simulink model "MCU_vectorControl_Simulation"  (R2024a)
settings: Solver=ode3  StartTime=0.0  StopTime=3  FixedStep=Ts  MaxStep=1e-4  RelTol=1e-3  EnableMultiTasking=on
values from neighbouring files (symbols this model uses):
  Ts = 1e-4    (= 0.0001)    [MCU_initVectorControlParameters.m]
undefined symbols (not defined in the file or in its folder): control, DiscIntNeverNeededParam, dspic33CK, insa_motormodel, inverter, LVMC, motor, NumBits1, NumBits2, PMSM, PosRange1, PosRange2, Slope1, Slope2
libraries: simulink x22, embmathops x1
(part 1 of 2)
Description:
  | Motor Control Simulation Demo
  | contacts : romain.delpoux@insa-lyon.fr, lubin.kerhuel@microchip.com
settings Model: DSRTSU_INTERNAL_RTI_VER=470  DSRTSU_INTERNAL_RTI_TYPE=rti1104  DSRTSU_INTERNAL_RTIFPGA=60  Creator=rdelpoux  LastModifiedBy=rdelpoux
settings SolverCC: ZeroCrossControl=DisableAll  AlgebraicLoopSolver=TrustRegion
settings DataIOCC: LimitDataPoints=on  SaveFormat=Array  ReturnWorkspaceOutputs=off
settings OptimizationCC: BlockReduction=off  OptimizeBlockIOStorage=off  BufferReuse=off  ReuseModelBlockBuffer=off  GlobalBufferReuse=off  ExpressionFolding=off  LocalBlockOutputs=off  LifeSpan=inf  OptimizeDataStoreBuffers=off  BusAssignmentInplaceUpdate=off
settings DebuggingCC: SolverPrmCheckMsg=warning  MultiTaskDSMMsg=none  UnconnectedInputMsg=warning  UnconnectedOutputMsg=warning  UnconnectedLineMsg=warning  SFUnexpectedBacktrackingDiag=warning  SFNoUnconditionalDefaultTransitionDiag=warning  SFExecutionAtInitializationDiag=none  ArithmeticOperatorsInVariantConditions=warning
settings HardwareCC: ProdBitPerPointer=32  ProdBitPerSizeT=32  ProdBitPerPtrDiffT=32  ProdLargestAtomicInteger=Integer  ProdEndianess=BigEndian  ProdWordSize=32  ProdHWDeviceType=Generic->Custom  TargetIntDivRoundTo=Zero  TargetEndianess=BigEndian  TargetHWDeviceType=Generic->Custom
settings ModelReferenceCC: EnableRefExpFcnMdlSchedulingChecks=on  PropagateSignalLabelsOutOfModel=off
settings SFSimCC: SimUseLocalCustomCode=off  CustomCodeUndefinedFunction=UseInterfaceOnly
settings RTWCC: Description=dSPACE DS1104 Hardware Platform  SystemTargetFile=rti1104.tlc  MakeCommand=make_rti  TemplateMakefile=rti1104.tmf  RTWUseLocalCustomCode=off  GPUComputeCapability=3.5  DLArmComputeVersion=19.05
settings CodeAppCC: StateflowObjectComments=on
settings STFCustomTargetCC: TargetLangStandard=C89/C90 (ANSI)  ParMdlRefBuildCompliant=on  MatFileLogging=on  UseToolchainInfoCompliant=off  SystemTargetFile=rti1104.tlc
settings GRTTargetCC: TargetLangStandard=C89/C90 (ANSI)  CompOptLevelCompliant=off  ConcurrentExecutionCompliant=off  CombineOutputUpdateFcns=off  CPPClassGenCompliant=off  GRTInterface=on  UseToolchainInfoCompliant=off  ExtModeMexFile=noextcomm
settings ConfigComp: CovMetricSettings=dw  CovSaveCumulativeToWorkspaceVar=on  CovSaveSingleToWorkspaceVar=on  CovExternalEMLEnable=off  CovSFcnEnable=off

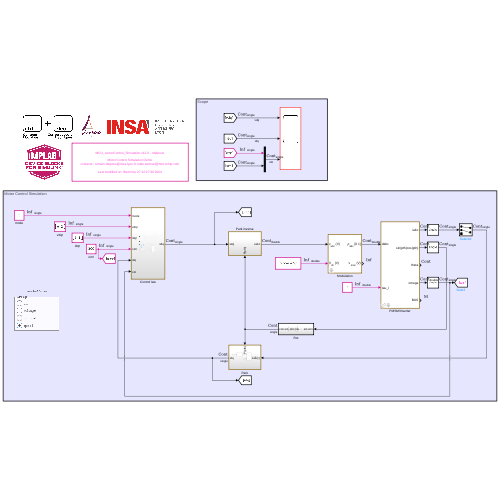
[thumbnail: Simulink's stored preview of the top-level diagram]
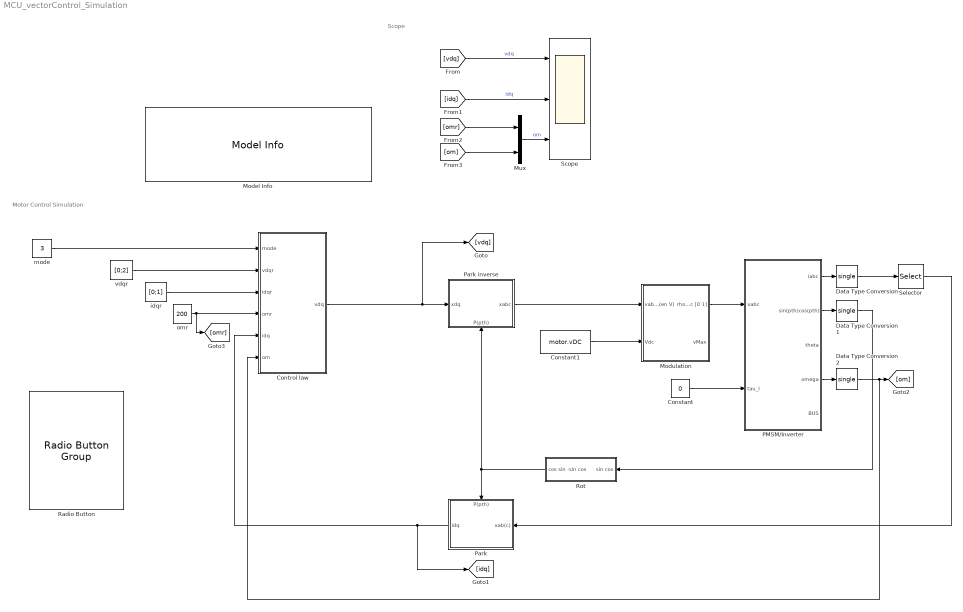
== system MCU_vectorControl_Simulation ==
  note: Scope
  note: Motor Control Simulation
  Constant : Constant  Value=0
  Constant1 : Constant  Value=motor.vDC
  Control law : Subsystem
      settings: LibrarySourceBlock=insa_control_base/Control law
  Data Type Conversion : DataTypeConversion  OutDataTypeStr=single  SaturateOnIntegerOverflow=off  RndMeth=Floor
  Data Type Conversion1 : DataTypeConversion  OutDataTypeStr=single  SaturateOnIntegerOverflow=off  RndMeth=Floor
  Data Type Conversion2 : DataTypeConversion  OutDataTypeStr=single  SaturateOnIntegerOverflow=off  RndMeth=Floor
  Model Info : simulink/Model-Wide Utilities/Model Info  Frame=on  DisplayStringWithTags=|  HorizontalTextAlignment=Center  LeftAlignmentValue=0.5
      | %<ModelName> v%<ModelVersion> - %<Creator>
      | 
      | %<Description>
      | 
      | Last modified on: %<LastModificationDate>
  Modulation : Subsystem  mask{modulation=Space Vector, mod=0}
      mask init:
      | switch modulation
      |     case 'Sinusoidale'
      |         mod = 0;
      |     otherwise
      |         mod = 1;
      | end
      mask TypeOptions modulation: Sinusoidale | Space Vector
      mask DialogControl DescGroupVar Prompt: Modulation interssecticve
      mask DialogControl DescTextVar Prompt: Choose between sinus or space vector modulation
      mask Display:
      | port_label('output', 1, '\rho_{abc} [0 1]', 'texmode','on')
      | port_label('output', 2, 'v_{\rm max} (V)', 'texmode','on')
      | port_label('input', 1, 'v_{abc} (V)', 'texmode','on')
      | port_label('input', 2, 'V_{dc} (V)', 'texmode','on')
  Mux : Mux  Inputs=2
  PMSM/Inverter : Subsystem  AncestorBlock=insa_motormodel/PMSM  mask(Test){presetMotor=Teknic-2310P, modelPMSM=Teknic-2310P, p=4, R=0.656, L=0.00035, Phif=0.0066, J=1e-05, F=1e-05, C0=0.01, omegaMax=350, encoderLines=1000, enableInverter=on, presetInverter=LVMC (DM330031), modelInverter=dspic33CK-LVMC, Vdc=24, iMax=10, FPWM=20000, PWMmax=5000, enableDTcomp=off, dT=1, ADCbits=12, ADCgainCurr=21.83, ADCgainVolt=69.3, Ts=1e-4}
      mask prompts: presetMotor "Pre Defined Motor"; modelPMSM "PMSM model"; p "Pole pairs p"; R "Phase resistor R (Ohm)"; L "Phase inductance L (H)"; Phif "Flux constant Phif (Wb)"; J "Inertia J (kg.m^2)"; F "Damping coefficient F (N.m.s/rad)"; C0 "Coulomb friction C0 (N.m)"; omegaMax "Max Speed (rad/s)"; encoderLines "lines"; enableInverter "Enable"; presetInverter "Pre Defined Inverter"; modelInverter "Inverter Model"; Vdc "DC Voltage Vdc (V)"; iMax "Max Current iMax (A)"; FPWM "PWM frequency"; enableDTcomp "Dead time Compensation"; dT "Dead time (us)"; ADCbits "Precision (bits)"; ADCgainCurr "Currents gain"; ADCgainVolt "Voltage gain"; Ts "Ts (s)"
      mask init:
      | % Mototor definition
      | pmsm = struct;
      | switch presetMotor
      |     case 'Teknic-2310P'
      |         pmsm.modelPMSM    = 'Teknic-2310P';                                     %           // Manufacturer Model Number
      |         pmsm.p        = 4;                                                  %           // Pole Pairs for the motor
      |         pmsm.R        = 0.656;                                              %Ohm        // Stator Resistor
      |         pmsm.L        = 0.35e-3;                                            %H          // Inductance value
      |         pmsm.Phif     = 6.6e-3;                                             %Wb         // PM flux
      |         pmsm.J        = 1e-05;                                              %Kg-m2      // Inertia in SI units
      |         pmsm.F        = 1.e-05;                                             %Kg-m2/s    // Friction Co-efficient
      |         pmsm.C0       = 0.01;                                               %Kg-m2      // Dry friction
      |         pmsm.omegaMax    = 350;                                            %rad/spm    // Max speed
      |         pmsm.encoderLines = 1000;
      |     case 'Custom'
      |         pmsm.modelPMSM    = 'Custom';                                           %           // Manufacturer Model Number
      |         pmsm.p        = p;                                                  %           // Pole Pairs for the motor
      |         pmsm.R        = R;                                                  %Ohm        // Stator Resistor
      |         pmsm.L        = L;                                                  %H          // Inductance value
      |         pmsm.Phif     = Phif;                                               %Wb         // PM flux
      |         pmsm.J        = J;                                                  %Kg-m2      // Inertia in SI units
      |         pmsm.F        = F;                                                  %Kg-m2/s    // Friction Co-efficient
      |         pmsm.C0       = C0;                                                 %Kg-m2      // Dry friction
      |         pmsm.omegaMax    = omegaMax;                                             %rad/spm    // Max speed
      |         pmsm.encoderLines = encoderLines;
      | end
      | 
      | ff = fields(pmsm);
      | for i=1:numel(ff)
      |     set_param(gcb,ff{i},num2str(pmsm.(ff{i})) );
      | end
      | 
      | % switch presetMotor
      | %      case 'Custom'
      | %          set_param(gcb,model,(pmsm.model) );
      | %      otherwise 'Teknic-2310P'
      | %
      | %
      | % end
      | 
      | assignin('base','pmsm',pmsm);
      | 
      | % Inverter Definition
      | inverter = struct;
      | switch presetInverter
      |     case 'LVMC (DM330031)'
      |         inverter.modelInverter = 'dspic33CK-LVMC';
      |         inverter.vDC = 24;                          %V          // DC voltage
      |         inverter.iMax = 10;                         %A      	// Rated current (phase-peak)
      |         inverter.ADCbits = 12;                      %bits       // ADC precision
      |         inverter.ADCgainCurr = 21.83;                   %
      |         inverter.ADCgainVolt = 69.3;                   %
      |         inverter.PWMmax = 5000;
      |         inverter.dT = 1;                            %us         // Deat Time
      |         inverter.FPWM = 20e3;                       %Hz         // PWM frequency
      |     case 'MCLV2 (DM330021-2)'
      | end
      | 
      | ff = fields(inverter);
      | for i=1:numel(ff)
      |     set_param(gcb,ff{i},num2str(inverter.(ff{i})) );
      | end
      | assignin('base','inverter',inverter);
      | 
      | assignin('base','Ts',Ts);
      settings: LibrarySourceBlock=insa_motormodel/PMSM
      mask Help: disp('{\itEquation:}  \alpha^2 + \beta^2 \rightarrow \gamma^2, \chi, \phi_3 = {\bfcool}', 'texmode','on')
      mask TypeOptions presetMotor: Custom | Teknic-2310P | Short HURST (AC300020) | Long HURST (AC300022)
      mask TypeOptions presetInverter: Custom | LVMC (DM330031) | MCLV2 (DM330021-2)
      mask DialogControl DescGroupVar Prompt: Moteur Synchrone à aimants permanents
      mask DialogControl DescTextVar Prompt: PMSM Model
      mask DialogControl Container6 Prompt: Motor Parameters
      mask DialogControl Container3 Prompt: Electrical parameters
      mask DialogControl Container4 Prompt: Mecanical parameter
      mask DialogControl Container9 Prompt: Encoder
      mask DialogControl Container11 Prompt: Inverter
      mask DialogControl Container12 Prompt: Inverter Constraints
      mask DialogControl Container10 Prompt: PWM
      mask DialogControl Container8 Prompt: ADC
      mask DialogControl Container13 Prompt: Sample Time
      mask Display:
      | switch get_param(gcb,'enableInverter')
      |     case 'off'
      |     port_label('input', 1, 'vabc');
      |     case 'on'
      |     port_label('input', 1, 'dabc');
      | end
      | port_label('input', 2, 'tau_l');
      | 
      | port_label('output', 1, 'iabc');
      | port_label('output', 2, 'sin(pth)cos(pth)');
      | port_label('output', 3, 'theta');
      | port_label('output', 4, 'omega');
      | port_label('output', 5, 'BUS');
  Park : Subsystem
      settings: PortSchema="{\"entries\":[{\"content\":{\"sides\":[{\"content\":{\"connectorIds\":[\"In1\"]},\"type\":\"ConnectorPlacement.EquallySpacedRectSide\",\"uuid\":\"ebf2fcb8-f94c-4630-a735-fb74e68b604e\"},{\"content\":{\"connectorIds\":[\"Out1\"],\"side\":\"RIGHT\"},\"type\":\"ConnectorPlacement.EquallySpacedRectSide\",\"uuid\":\"fb89ad3f-9420-4065-992c-c6d77ce245e0\"},{\"content\":{\"connectorIds\":[\"In2\"],\"side\":\"TOP\"},\"type\":\"ConnectorPlacement.EquallySpacedRectSide\",\"uuid\":\"0249ceba-2241-48c9-87d4-d9d6f381f2d7\"}]},\"type\":\"ConnectorPlacement.EquallySpacedConnector\",\"uuid\":\"eecfd82d-5918-403e-a677-09fe1d8cc737\"}],\"packageUris\":[\"http://schema.mathworks.com/mf0/Connector/R2020b\"],\"version\":\"1.0\"}"
  Park inverse : Subsystem
      settings: PortSchema="{\"entries\":[{\"content\":{\"sides\":[{\"content\":{\"connectorIds\":[\"In1\"]},\"type\":\"ConnectorPlacement.EquallySpacedRectSide\",\"uuid\":\"4c11ef0a-1978-4a73-9b5c-4d5650fcee33\"},{\"content\":{\"connectorIds\":[\"Out1\"],\"side\":\"RIGHT\"},\"type\":\"ConnectorPlacement.EquallySpacedRectSide\",\"uuid\":\"28284572-70c7-45ef-9db5-4b5788e96454\"},{\"content\":{\"side\":\"TOP\"},\"type\":\"ConnectorPlacement.EquallySpacedRectSide\",\"uuid\":\"3a1fbce2-0868-491b-8e3a-2b3a7a0d615d\"},{\"content\":{\"connectorIds\":[\"In2\"],\"side\":\"BOTTOM\"},\"type\":\"ConnectorPlacement.EquallySpacedRectSide\",\"uuid\":\"e63426ef-821a-4774-a922-a3f70d9b2116\"}]},\"type\":\"ConnectorPlacement.EquallySpacedConnector\",\"uuid\":\"285593a5-8af6-47f2-83d9-d6ebce98de71\"}],\"packageUris\":[\"http://schema.mathworks.com/mf0/Connector/R2020b\"],\"version\":\"1.0\"}"
  Radio Button : RadioButtonGroup  SelectedLabel=speed  ButtonGroupName=Group
      settings: Values={{'off', 'voltage', 'current', 'speed'}, [0 1 2 3]}
  Rot : Subsystem
  Scope : Scope  NumInputPorts=3
  Selector : Selector  InputPortWidth=3  IndexOptions=Index vector (dialog)  Indices=[1 2]  OutputSizes=1
  idqr : Constant  Value=[0;1]  OutDataTypeStr=single
  mode : Constant  Value=3  OutDataTypeStr=single
  omr : Constant  Value=200  OutDataTypeStr=single
  vdqr : Constant  Value=[0;2]  OutDataTypeStr=single
  wires:
  [vdq] -> Scope/1  "vdq"
  [idq] -> Scope/2  "idq"
  [omr] -> Mux/1
  [om] -> Mux/2
  Mux/1 -> Scope/3  "om"
  Control law/1(vdq) -> [vdq], Park inverse/1(xdq)
  vdqr/1 -> Control law/2(vdqr)
  mode/1 -> Control law/1(mode)
  omr/1 -> Control law/4(omr), [omr]
  idqr/1 -> Control law/3(idqr)
  Constant/1 -> PMSM/Inverter/2(tau_l)
  PMSM/Inverter/1(iabc) -> Data Type Conversion/1
  Selector/1 -> Park/1(xab(c))
  PMSM/Inverter/2(sin(pth)cos(pth)) -> Data Type Conversion1/1
  Modulation/1(rho_abc [0 1]) -> PMSM/Inverter/1(xabc)
  PMSM/Inverter/4(omega) -> Data Type Conversion2/1
  Park/1(idq) -> Control law/5(idq), [idq]
  Data Type Conversion/1 -> Selector/1
  Data Type Conversion1/1 -> Rot/1(sin cos)
  Data Type Conversion2/1 -> Control law/6(om), [om]
  Constant1/1 -> Modulation/2(Vdc)
  Rot/1("cos sin -sin cos ") -> Park inverse/2(P(pth)), Park/2(P(pth))
  Park inverse/1(xabc) -> Modulation/1("vabc (en V) ")

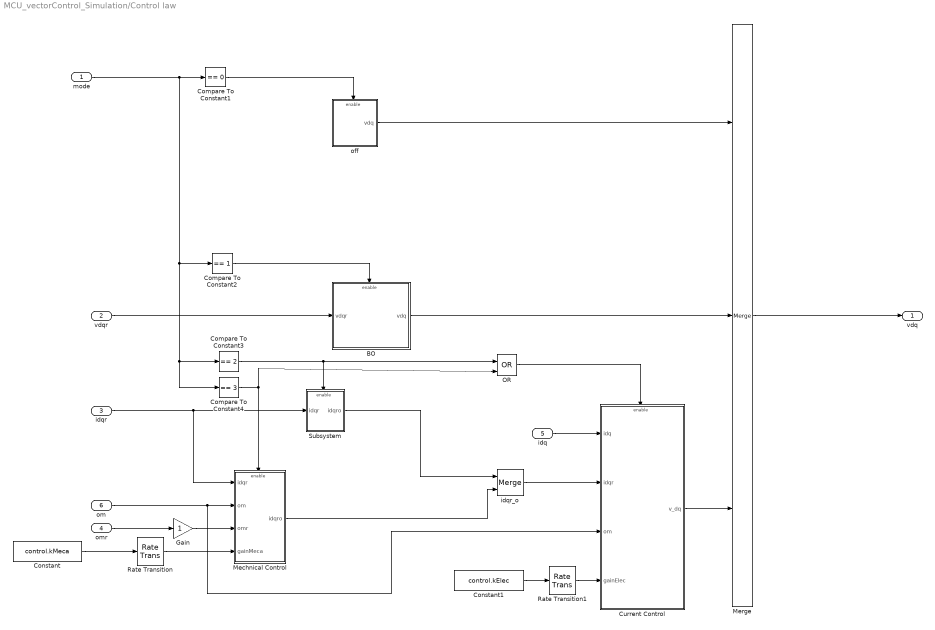
== system MCU_vectorControl_Simulation/Control law ==
  mode : Inport
  vdqr : Inport  Port=2
  idqr : Inport  Port=3
  omr : Inport  Port=4
  idq : Inport  Port=5
  om : Inport  Port=6
  BO : Subsystem
  Compare To Constant1 : simulink/Logic and Bit Operations/Compare To Constant  relop===  const=0  OutDataTypeStr=boolean
  Compare To Constant2 : simulink/Logic and Bit Operations/Compare To Constant  relop===  const=1  OutDataTypeStr=boolean
  Compare To Constant3 : simulink/Logic and Bit Operations/Compare To Constant  relop===  const=2  OutDataTypeStr=boolean
  Compare To Constant4 : simulink/Logic and Bit Operations/Compare To Constant  relop===  const=3  OutDataTypeStr=boolean
  Constant : Constant  Value=control.kMeca  OutDataTypeStr=single
  Constant1 : Constant  Value=control.kElec  OutDataTypeStr=double
  Current Control : Subsystem  AncestorBlock=insa_control_base/Current Control
      settings: LibrarySourceBlock=insa_control_base/Current Control
  Gain : Gain
  Mechnical Control : Subsystem
  Merge : Merge  Inputs=3
  OR : Logic  Operator=OR  IconShape=distinctive  AllPortsSameDT=off  OutDataTypeStr=boolean
  Rate Transition : RateTransition
  Rate Transition1 : RateTransition
  Subsystem : Subsystem
  idqr_o : Merge
  off : Subsystem
  vdq : Outport  VectorParamsAs1DForOutWhenUnconnected=off
  wires:
  omr/1 -> Gain/1
  idqr/1 -> Mechnical Control/1(idqr), Subsystem/1(idqr)
  vdqr/1 -> BO/1(vdqr)
  Current Control/1(v_dq) -> Merge/3
  idqr_o/1 -> Current Control/2(idqr)
  idq/1 -> Current Control/1(idq)
  OR/1 -> Current Control/Enable
  om/1 -> Current Control/3(om), Mechnical Control/2(om)
  Compare To Constant4/1 -> Mechnical Control/Enable, OR/2
  Mechnical Control/1(idqro) -> idqr_o/2
  Subsystem/1(idqro) -> idqr_o/1
  mode/1 -> Compare To Constant1/1, Compare To Constant4/1, Compare To Constant3/1, Compare To Constant2/1
  Compare To Constant3/1 -> Subsystem/Enable, OR/1
  Compare To Constant1/1 -> off/Enable
  off/1(vdq) -> Merge/1
  Compare To Constant2/1 -> BO/Enable
  BO/1(vdq) -> Merge/2
  Merge/1 -> vdq/1
  Constant/1 -> Rate Transition/1
  Constant1/1 -> Rate Transition1/1
  Rate Transition/1 -> Mechnical Control/4(gainMeca)
  Rate Transition1/1 -> Current Control/4(gainElec)
  Gain/1 -> Mechnical Control/3(omr)

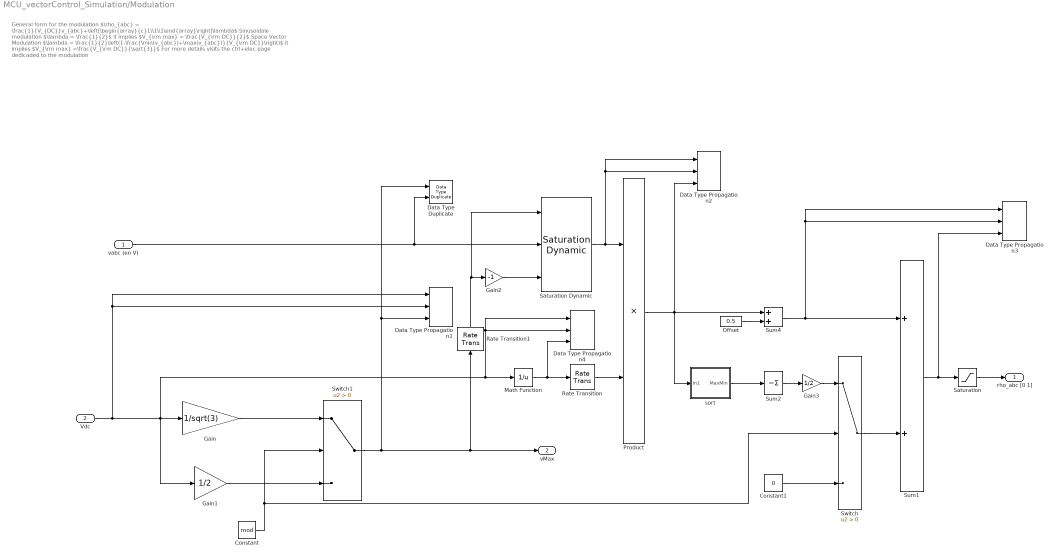
== system MCU_vectorControl_Simulation/Modulation ==
  note: General form for the modulation
      | $\rho_{abc} = \frac{1}{V_{DC}}v_{abc}+\left[\begin{array}{c}1\\1\\1\end{array}\right]\lambda$
      | Sinusoidale modulation
      | $\lambda = \frac{1}{2}$ it implies $V_{\rm max} = \frac{V_{\rm DC}}{2}$
      | Space Vector Modulation
      | $\lambda = \frac{1}{2}\left(1-\frac{\min(v_{abc})+\max(v_{abc})}{V_{\rm DC}}\right)$ it implies $V_{\rm max} =\frac{V_{\rm DC}}{\sqrt{3}}$
      | For more details visits the ctrl+elec page dedicaded to the modulation
  "vabc (en V) " : Inport
  Vdc : Inport  Port=2
  Constant : Constant  Value=mod  OutDataTypeStr=boolean
  Constant1 : Constant  Value=0  OutDataTypeStr=Inherit: Inherit via back propagation
  Data Type Duplicate : DataTypeDuplicate
  Data Type Propagation1 : simulink/Signal Attributes/Data Type Propagation  PropDataType=fixdt(1, 16)  IfRefDouble=double  IfRefSingle=single  IsSigned=TRUE  NumBitsBase=max([NumBits1 NumBits2])  NumBitsMult=1  NumBitsAdd=0  NumBitsAllowFinal=[1:128]  PropScaling=2^-(15-ceil(log2(inverter.vDC/sqrt(3))))  ValuesUsedBestPrec=[100 -100]  SlopeBase=max([PosRange1 PosRange2])  SlopeMult=1/sqrt(3)  SlopeAdd=0  BiasBase=Bias1  BiasMult=1  BiasAdd=0
  Data Type Propagation2 : simulink/Signal Attributes/Data Type Propagation  PropDataType=fixdt(1, 16)  IfRefDouble=double  IfRefSingle=single  IsSigned=TRUE  NumBitsBase=max([NumBits1 NumBits2])  NumBitsMult=1  NumBitsAdd=0  NumBitsAllowFinal=[1:128]  PropScalingMode=Specify via dialog  PropScaling=2^-14  ValuesUsedBestPrec=[100 -100]  SlopeBase=Slope1/Slope2  SlopeMult=1  SlopeAdd=0  BiasBase=Bias1  BiasMult=1  BiasAdd=0
  Data Type Propagation3 : simulink/Signal Attributes/Data Type Propagation  PropDataType=fixdt(1, 16)  IfRefDouble=double  IfRefSingle=single  IsSigned=FALSE  NumBitsBase=max([NumBits1 NumBits2])  NumBitsMult=1  NumBitsAdd=0  NumBitsAllowFinal=[1:128]  PropScalingMode=Specify via dialog  PropScaling=2^-14  ValuesUsedBestPrec=[100 -100]  SlopeBase=Slope1/Slope2  SlopeMult=1  SlopeAdd=0  BiasBase=Bias1  BiasMult=1  BiasAdd=0
  Data Type Propagation4 : simulink/Signal Attributes/Data Type Propagation  PropDataType=fixdt(1, 16)  IfRefDouble=double  IfRefSingle=single  IsSigned=FALSE  NumBitsBase=max([NumBits1 NumBits2])  NumBitsMult=1  NumBitsAdd=0  NumBitsAllowFinal=[1:128]  PropScalingMode=Specify via dialog  PropScaling=2^-16  ValuesUsedBestPrec=[100 -100]  SlopeBase=max([PosRange1 PosRange2])  SlopeMult=1/sqrt(3)  SlopeAdd=0  BiasBase=Bias1  BiasMult=1  BiasAdd=0
  Gain : Gain  Gain=1/sqrt(3)  OutDataTypeStr=Inherit: Same as input
  Gain1 : Gain  Gain=1/2  OutDataTypeStr=Inherit: Same as input
  Gain2 : Gain  Gain=-1  ParamDataTypeStr=int16  OutDataTypeStr=Inherit: Inherit via back propagation
  Gain3 : Gain  Gain=1/2  OutDataTypeStr=Inherit: Same as input
  Math Function : Math  Operator=reciprocal  OutputSignalType=real  OutDataTypeStr=Inherit: Inherit via back propagation  SaturateOnIntegerOverflow=off
  "Offset " : Constant  Value=0.5  OutMin=[0]  OutMax=[1]  OutDataTypeStr=Inherit: Inherit via back propagation
  Product : Product  Inputs=**  OutDataTypeStr=Inherit: Inherit via back propagation  SaturateOnIntegerOverflow=on
  Rate Transition : RateTransition
  Rate Transition1 : RateTransition
  Saturation : Saturate  UpperLimit=1  LowerLimit=0
  Saturation Dynamic : simulink/Discontinuities/Saturation Dynamic  OutMin=[]  OutMax=[]  OutDataTypeStr=Inherit: Same as second input  OutDataType=fixdt(1, 16)  OutScaling=2^-10  DoSatur=off
  Sum1 : Sum  OutMin=[0]  OutMax=[1]  OutDataTypeStr=Inherit: Inherit via back propagation  InputSameDT=on  SaturateOnIntegerOverflow=on
  Sum2 : Sum  Inputs=-  OutMin=[-1]  OutMax=[1]  InputSameDT=on  SaturateOnIntegerOverflow=on  OutDataTypeStr=Inherit: Same as first input
  Sum4 : Sum  OutMin=[-1]  OutMax=[1]  InputSameDT=on  SaturateOnIntegerOverflow=on  OutDataTypeStr=Inherit: Same as first input
  Switch : Switch  Criteria=u2 > Threshold  SaturateOnIntegerOverflow=off  InputSameDT=off
  Switch1 : Switch  Criteria=u2 > Threshold  OutDataTypeStr=Inherit: Inherit via back propagation  SaturateOnIntegerOverflow=off  InputSameDT=off
  sort : Subsystem
  rho_abc [0 1] : Outport  VectorParamsAs1DForOutWhenUnconnected=off
  vMax : Outport  Port=2  VectorParamsAs1DForOutWhenUnconnected=off
  wires:
  Sum1/1 -> Saturation/1, Data Type Propagation3/3
  Vdc/1 -> Data Type Propagation1/2, Data Type Propagation1/1, Gain/1, Math Function/1, Data Type Propagation4/2, Data Type Propagation4/1, Gain1/1
  Gain3/1 -> Switch/1
  Saturation/1 -> rho_abc [0 1]/1
  Saturation Dynamic/1 -> Product/1, Data Type Propagation2/1, Data Type Propagation2/2
  Gain1/1 -> Switch1/3
  Gain/1 -> Switch1/1
  sort/1(MaxMin) -> Sum2/1
  Sum2/1 -> Gain3/1
  Sum4/1 -> Data Type Propagation3/2, Data Type Propagation3/1, Sum1/1
  Constant1/1 -> Switch/3
  Switch/1 -> Sum1/2
  "Offset "/1 -> Sum4/2
  Product/1 -> Data Type Propagation2/3, Sum4/1, sort/1(In1)
  Gain2/1 -> Saturation Dynamic/3
  Math Function/1 -> Data Type Propagation4/3, Rate Transition/1
  Switch1/1 -> Rate Transition1/1, vMax/1, Data Type Propagation1/3, Data Type Duplicate/1
  Constant/1 -> Switch1/2, Switch/2
  "vabc (en V) "/1 -> Data Type Duplicate/2, Saturation Dynamic/2
  Rate Transition/1 -> Product/2
  Rate Transition1/1 -> Saturation Dynamic/1, Gain2/1

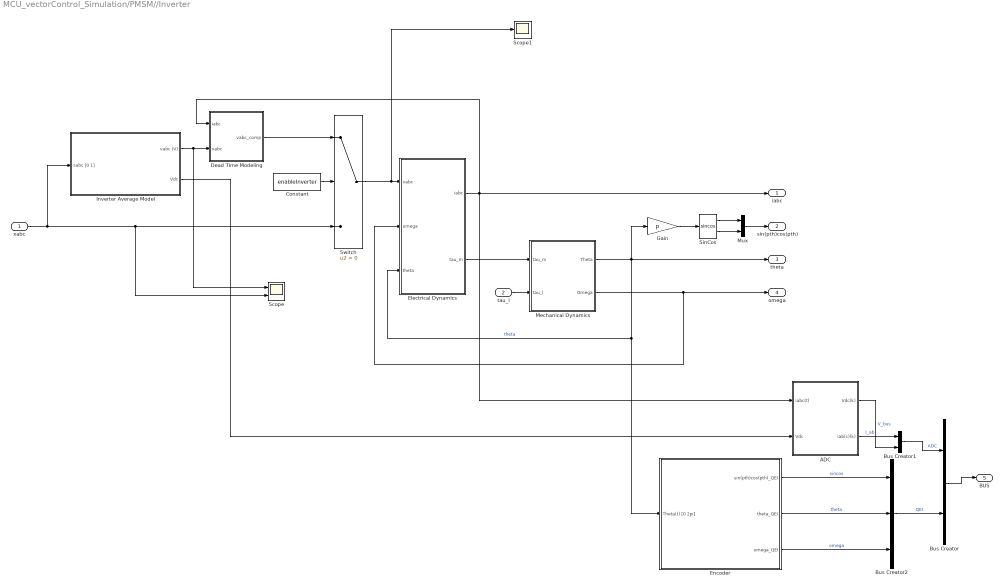
== system MCU_vectorControl_Simulation/PMSM//Inverter ==
  xabc : Inport
  tau_l : Inport  Port=2
  ADC : Subsystem
  Bus Creator : BusCreator  Inputs=2
  Bus Creator1 : BusCreator  Inputs=2
  Bus Creator2 : BusCreator  Inputs=3
  Constant : Constant  Value=enableInverter  OutDataTypeStr=boolean
  Dead Time Modeling : Subsystem
  Electrical Dynamics : Subsystem
  Encoder : Subsystem
  Gain : Gain  Gain=p
  Inverter Average Model : Subsystem
      settings: LibrarySourceBlock=insa_motormodel/Inverter Average Model
  Mechanical Dynamics : Subsystem
  Mux : Mux  Inputs=2
  Scope : Scope  NumInputPorts=2
  Scope1 : Scope
  SinCos : Trigonometry  Operator=sincos
  Switch : Switch  Criteria=u2 > Threshold  SaturateOnIntegerOverflow=off  InputSameDT=off
  iabc : Outport  VectorParamsAs1DForOutWhenUnconnected=off
  sin(pth)cos(pth) : Outport  Port=2  VectorParamsAs1DForOutWhenUnconnected=off
  theta : Outport  Port=3  VectorParamsAs1DForOutWhenUnconnected=off
  omega : Outport  Port=4  VectorParamsAs1DForOutWhenUnconnected=off
  BUS : Outport  Port=5  VectorParamsAs1DForOutWhenUnconnected=off
  wires:
  xabc/1 -> Inverter Average Model/1(sabc [0 1]), Scope/2, Switch/3
  tau_l/1 -> Mechanical Dynamics/2(tau_l)
  Electrical Dynamics/1(iabc) -> Dead Time Modeling/1(iabc), ADC/1(iabc(t)), iabc/1
  Mechanical Dynamics/2(Omega) -> omega/1, Electrical Dynamics/2(omega)
  Electrical Dynamics/2(tau_m) -> Mechanical Dynamics/1(tau_m)
  SinCos/2 -> Mux/2
  Mux/1 -> sin(pth)cos(pth)/1
  SinCos/1 -> Mux/1
  Gain/1 -> SinCos/1
  Mechanical Dynamics/1(Theta) -> Gain/1, theta/1, Encoder/1(Theta(t) [0 2pi]), Electrical Dynamics/3(theta)  "theta"
  Bus Creator/1 -> BUS/1
  ADC/2(iab(c)(k)) -> Bus Creator1/1  "I_ab"
  Encoder/3(omega_QEI) -> Bus Creator2/3  "omega"
  Encoder/2(theta_QEI) -> Bus Creator2/2  "theta"
  Encoder/1(sin(pth)cos(pth)_QEI) -> Bus Creator2/1  "sincos"
  Inverter Average Model/1("vabc (V) ") -> Scope/1, Dead Time Modeling/2(vabc)
  Dead Time Modeling/1(vabc_comp) -> Switch/1
  Constant/1 -> Switch/2
  ADC/1(Vdc(k)) -> Bus Creator1/2  "V_bus"
  Inverter Average Model/2(Vdc) -> ADC/2(Vdc)
  Switch/1 -> Scope1/1, Electrical Dynamics/1(vabc)
  Bus Creator1/1 -> Bus Creator/1  "ADC"
  Bus Creator2/1 -> Bus Creator/2  "QEI"

== system MCU_vectorControl_Simulation/Park ==
  xab(c) : Inport
  P(pth) : Inport  Port=2
  Clarke : Subsystem
  Park : Subsystem
  idq : Outport
  wires:
  Clarke/1(xalphabeta) -> Park/1(xalphabeta)
  xab(c)/1 -> Clarke/1(xab(c))
  P(pth)/1 -> Park/2(P(pth))
  Park/1(xdq) -> idq/1  "idq"

== system MCU_vectorControl_Simulation/Park inverse ==
  xdq : Inport
  P(pth) : Inport  Port=2
  Clarke Inverse : Subsystem
  Park inverse : Subsystem
  xabc : Outport
  wires:
  P(pth)/1 -> Park inverse/2(P(pth))
  Clarke Inverse/1(xabc) -> xabc/1
  xdq/1 -> Park inverse/1(xdq)
  Park inverse/1(xalpahbeta) -> Clarke Inverse/1(xalphabeta)

== system MCU_vectorControl_Simulation/Rot ==
  sin cos : Inport
  Demux3 : Demux  Outputs=2
  Gain : Gain  Gain=-1  OutDataTypeStr=Inherit: Same as input
  Mux1 : Mux
  Reshape : Reshape  OutputDimensionality=Customize  OutputDimensions=[2,2]
  "cos sin -sin cos " : Outport  PortDimensions=[2 2]
  wires:
  Demux3/2 -> Mux1/1, Mux1/4
  Demux3/1 -> Gain/1, Mux1/3
  Mux1/1 -> Reshape/1
  Gain/1 -> Mux1/2
  sin cos/1 -> Demux3/1
  Reshape/1 -> "cos sin -sin cos "/1

== system MCU_vectorControl_Simulation/Control law/BO ==
  vdqr : Inport
  Enable : EnablePort
  vdq : Outport  VectorParamsAs1DForOutWhenUnconnected=off
  wires:
  vdqr/1 -> vdq/1

== system MCU_vectorControl_Simulation/Control law/Current Control ==
  idq : Inport
  idqr : Inport  Port=2
  om : Inport  Port=3
  gainElec : Inport  Port=4
  Enable : EnablePort  StatesWhenEnabling=reset
  Constant : Constant  Value=motor.p  OutDataTypeStr=single
  Constant1 : Constant  Value=motor.L  OutDataTypeStr=single
  Constant2 : Constant  Value=motor.Phif  OutDataTypeStr=single
  Current : Subsystem
  Voltage Saturation : Subsystem
  feedback lineazation : Subsystem
  v_dq : Outport
  wires:
  om/1 -> feedback lineazation/3(om)
  Voltage Saturation/1(vdqsat) -> v_dq/1
  idqr/1 -> Current/2(iqr)
  Current/1(v_dq) -> feedback lineazation/1(udq)
  idq/1 -> feedback lineazation/2(idq), Current/1(idq)
  gainElec/1 -> Current/4(Ke)
  Voltage Saturation/2(saturation) -> Current/3(saturation)
  feedback lineazation/1(v_dq) -> Voltage Saturation/1(vdq)
  Constant/1 -> feedback lineazation/4(p)
  Constant2/1 -> feedback lineazation/6(Phif)
  Constant1/1 -> feedback lineazation/5(L)

== system MCU_vectorControl_Simulation/Control law/Mechnical Control ==
  idqr : Inport
  om : Inport  Port=2
  omr : Inport  Port=3
  gainMeca : Inport  Port=4
  Enable : EnablePort  StatesWhenEnabling=reset
  Augmented state feedback : Subsystem
  Mux : Mux  Inputs=2
  Selector : Selector  InputPortWidth=2  IndexOptions=Index vector (dialog)  Indices=1  OutputSizes=1
  idqro : Outport  VectorParamsAs1DForOutWhenUnconnected=off
  wires:
  om/1 -> Augmented state feedback/2(om)
  Augmented state feedback/1(iqref) -> Mux/2
  omr/1 -> Augmented state feedback/1(omref)
  gainMeca/1 -> Augmented state feedback/3(gainMeca)
  idqr/1 -> Selector/1
  Mux/1 -> idqro/1
  Selector/1 -> Mux/1

== system MCU_vectorControl_Simulation/Control law/Subsystem ==
  idqr : Inport
  Enable : EnablePort
  idqro : Outport
  wires:
  idqr/1 -> idqro/1

== system MCU_vectorControl_Simulation/Control law/off ==
  Enable : EnablePort
  Mux : Mux  Inputs=2
  vd : Constant  Value=0  OutDataTypeStr=single
  vq : Constant  Value=0  OutDataTypeStr=single
  vdq : Outport  VectorParamsAs1DForOutWhenUnconnected=off
  wires:
  vd/1 -> Mux/1
  Mux/1 -> vdq/1
  vq/1 -> Mux/2

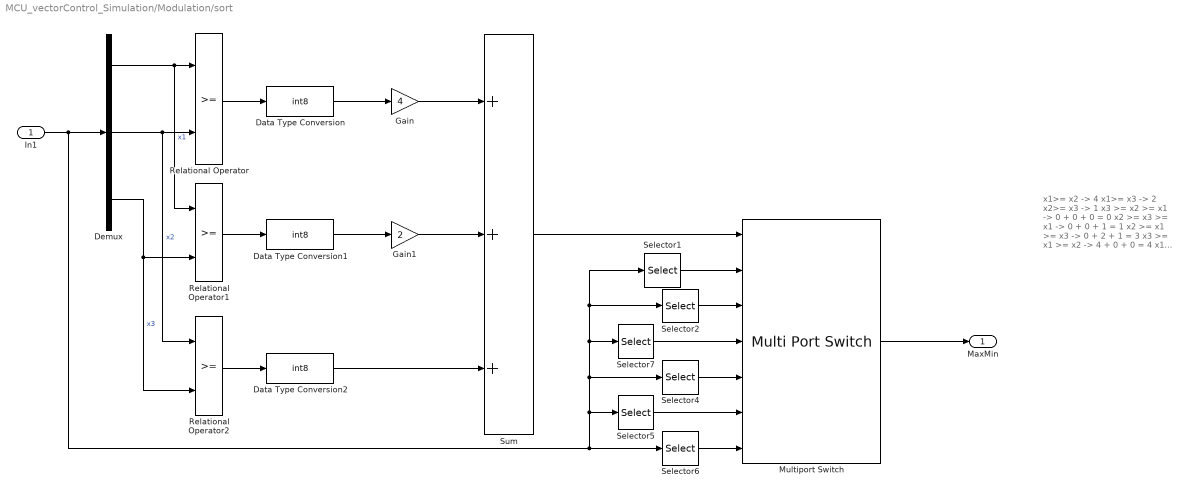
== system MCU_vectorControl_Simulation/Modulation/sort ==
  note: x1>= x2 -> 4
      | x1>= x3 -> 2
      | x2>= x3 -> 1
      |
      | x3 >= x2 >= x1 -> 0 + 0 + 0 = 0
      | x2 >= x3 >= x1 -> 0 + 0 + 1 = 1
      | x2 >= x1 >= x3 -> 0 + 2 + 1 = 3
      | x3 >= x1 >= x2 -> 4 + 0 + 0 = 4
      | x1 >= x3 >= x2 -> 4 + 2 + 0 = 6
      | x1 >= x2 >= x3 -> 4 + 2 + 1 = 7
  In1 : Inport
  Data Type Conversion : DataTypeConversion  OutDataTypeStr=int8  SaturateOnIntegerOverflow=off  RndMeth=Floor
  Data Type Conversion1 : DataTypeConversion  OutDataTypeStr=int8  SaturateOnIntegerOverflow=off  RndMeth=Floor
  Data Type Conversion2 : DataTypeConversion  OutDataTypeStr=int8  SaturateOnIntegerOverflow=off  RndMeth=Floor
  Demux : Demux  Outputs=3
  Gain : Gain  Gain=4  OutDataTypeStr=Inherit: Same as input
  Gain1 : Gain  Gain=2  OutDataTypeStr=Inherit: Same as input
  Multiport Switch : MultiPortSwitch  DataPortOrder=Specify indices  DataPortIndices={0,1,3,4,6,7}  SaturateOnIntegerOverflow=off  InputSameDT=off
  Relational Operator : RelationalOperator  OutDataTypeStr=boolean  RndMeth=Simplest  InputSameDT=off
  Relational Operator1 : RelationalOperator  OutDataTypeStr=boolean  RndMeth=Simplest  InputSameDT=off
  Relational Operator2 : RelationalOperator  OutDataTypeStr=boolean  RndMeth=Simplest  InputSameDT=off
  Selector1 : Selector  InputPortWidth=3  IndexOptions=Index vector (dialog)  Indices=[3 1]  OutputSizes=1
  Selector2 : Selector  InputPortWidth=3  IndexOptions=Index vector (dialog)  Indices=[2 1]  OutputSizes=1
  Selector4 : Selector  InputPortWidth=3  IndexOptions=Index vector (dialog)  Indices=[3 2]  OutputSizes=1
  Selector5 : Selector  InputPortWidth=3  IndexOptions=Index vector (dialog)  Indices=[1 2]  OutputSizes=1
  Selector6 : Selector  InputPortWidth=3  IndexOptions=Index vector (dialog)  Indices=[1 3]  OutputSizes=1
  Selector7 : Selector  InputPortWidth=3  IndexOptions=Index vector (dialog)  Indices=[2 3]  OutputSizes=1
  Sum : Sum  Inputs=+++
  MaxMin : Outport
  wires:
  Demux/3 -> Relational Operator2/2, Relational Operator1/2  "x3"
  Demux/2 -> Relational Operator2/1, Relational Operator/2  "x2"
  Demux/1 -> Relational Operator1/1, Relational Operator/1  "x1"
  In1/1 -> Selector4/1, Selector7/1, Selector2/1, Selector1/1, Selector5/1, Selector6/1, Demux/1
  Relational Operator2/1 -> Data Type Conversion2/1
  Relational Operator1/1 -> Data Type Conversion1/1
  Relational Operator/1 -> Data Type Conversion/1
  Data Type Conversion/1 -> Gain/1
  Data Type Conversion1/1 -> Gain1/1
  Gain1/1 -> Sum/2
  Gain/1 -> Sum/1
  Data Type Conversion2/1 -> Sum/3
  Sum/1 -> Multiport Switch/1
  Selector1/1 -> Multiport Switch/2
  Selector6/1 -> Multiport Switch/7
  Selector5/1 -> Multiport Switch/6
  Selector4/1 -> Multiport Switch/5
  Selector7/1 -> Multiport Switch/4
  Selector2/1 -> Multiport Switch/3
  Multiport Switch/1 -> MaxMin/1

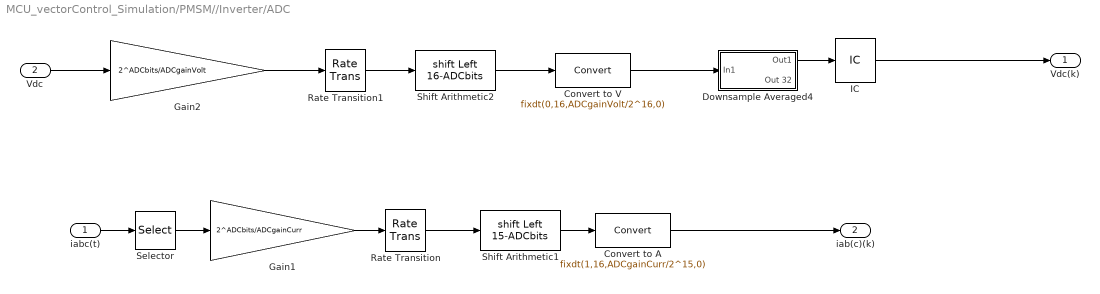
== system MCU_vectorControl_Simulation/PMSM//Inverter/ADC ==
  iabc(t) : Inport
  Vdc : Inport  Port=2
  Convert to A : DataTypeConversion  OutDataTypeStr=fixdt(1,16,ADCgainCurr/2^15,0)  ConvertRealWorld=Stored Integer (SI)  SaturateOnIntegerOverflow=off  RndMeth=Floor
  Convert to V : DataTypeConversion  OutDataTypeStr=fixdt(0,16,ADCgainVolt/2^16,0)  ConvertRealWorld=Stored Integer (SI)  SaturateOnIntegerOverflow=off  RndMeth=Floor
  Downsample Averaged4 : Subsystem  mask{DownSample=20}
      mask prompts: DownSample "DownSample Factor"
  Gain1 : Gain  Gain=2^ADCbits/ADCgainCurr  OutDataTypeStr=int16
  Gain2 : Gain  Gain=2^ADCbits/ADCgainVolt  OutDataTypeStr=int16
  IC : InitialCondition  Value=Vdc
  Rate Transition : RateTransition  OutPortSampleTime=Ts
  Rate Transition1 : RateTransition  OutPortSampleTime=Ts
  Selector : Selector  InputPortWidth=3  IndexOptions=Index vector (dialog)  Indices=[1 2]  OutputSizes=1
  Shift Arithmetic1 : ArithShift  BitShiftNumber=15-ADCbits  BitShiftDirection=Left
  Shift Arithmetic2 : ArithShift  BitShiftNumber=16-ADCbits  BitShiftDirection=Left
  Vdc(k) : Outport
  iab(c)(k) : Outport  Port=2
  wires:
  Convert to A/1 -> iab(c)(k)/1
  Selector/1 -> Gain1/1
  iabc(t)/1 -> Selector/1
  Gain1/1 -> Rate Transition/1
  Shift Arithmetic1/1 -> Convert to A/1
  Rate Transition/1 -> Shift Arithmetic1/1
  Vdc/1 -> Gain2/1
  Rate Transition1/1 -> Shift Arithmetic2/1
  Shift Arithmetic2/1 -> Convert to V/1
  Gain2/1 -> Rate Transition1/1
  Convert to V/1 -> Downsample Averaged4/1(In1)
  Downsample Averaged4/1(Out1) -> IC/1
  IC/1 -> Vdc(k)/1

== system MCU_vectorControl_Simulation/PMSM//Inverter/Dead Time Modeling ==
  note: $v_{abc,{\rm comp}} = v_{abc}-\Delta v_{abc}\\ \Delta v_{abc} = \frac{dT}{T_{\rm PWM}}.V_{\rm DC}.\text{sign}(i_{abc})$
  iabc : Inport
  vabc : Inport  Port=2
  Constant : Constant  Value=enableDTcomp  OutDataTypeStr=boolean
  Constant1 : Constant  Value=0
  DeadTime Compensation : Subsystem
  Sum : Sum  Inputs=-+|
  Switch : Switch  Criteria=u2 > Threshold  SaturateOnIntegerOverflow=off  InputSameDT=off
  vabc_comp : Outport
  wires:
  Switch/1 -> Sum/1
  Sum/1 -> vabc_comp/1
  vabc/1 -> Sum/2
  Constant/1 -> Switch/2, DeadTime Compensation/Enable
  DeadTime Compensation/1(Delta vabc) -> Switch/1
  iabc/1 -> DeadTime Compensation/1(iabc)
  Constant1/1 -> Switch/3

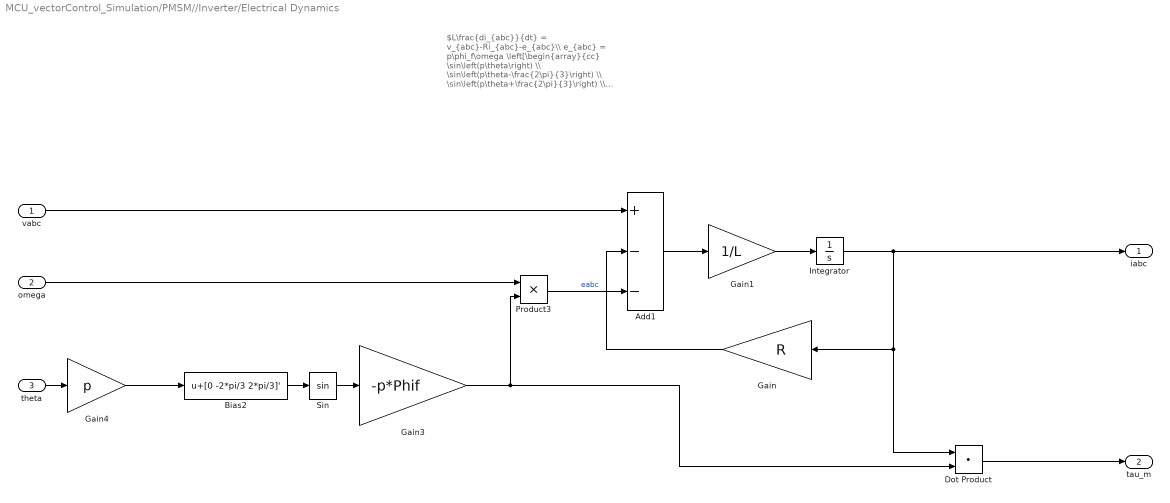
== system MCU_vectorControl_Simulation/PMSM//Inverter/Electrical Dynamics ==
  note: $L\frac{di_{abc}}{dt} = v_{abc}-Ri_{abc}-e_{abc}\\ e_{abc} = p\phi_f\omega \left[\begin{array}{cc} \sin\left(p\theta\right) \\ \sin\left(p\theta-\frac{2\pi}{3}\right) \\ \sin\left(p\theta+\frac{2\pi}{3}\right) \\ \end{array}\right]$
  vabc : Inport
  omega : Inport  Port=2
  theta : Inport  Port=3
  Add1 : Sum  Inputs=+--
  Bias2 : Bias  Bias=[0 -2*pi/3 2*pi/3]'  SaturateOnIntegerOverflow=off
  Dot Product : DotProduct  OutDataTypeStr=Inherit: Inherit via internal rule
  Gain : Gain  Gain=R
  Gain1 : Gain  Gain=1/L
  Gain3 : Gain  Gain=-p*Phif
  Gain4 : Gain  Gain=p
  Integrator : Integrator
  Product3 : Product
  Sin : Trigonometry
  iabc : Outport  VectorParamsAs1DForOutWhenUnconnected=off
  tau_m : Outport  Port=2  VectorParamsAs1DForOutWhenUnconnected=off
  wires:
  Integrator/1 -> Dot Product/1, Gain/1, iabc/1
  Add1/1 -> Gain1/1
  vabc/1 -> Add1/1
  Gain/1 -> Add1/2
  Gain1/1 -> Integrator/1
  theta/1 -> Gain4/1
  Dot Product/1 -> tau_m/1
  Product3/1 -> Add1/3  "eabc"
  omega/1 -> Product3/1
  Bias2/1 -> Sin/1
  Gain3/1 -> Product3/2, Dot Product/2
  Gain4/1 -> Bias2/1
  Sin/1 -> Gain3/1

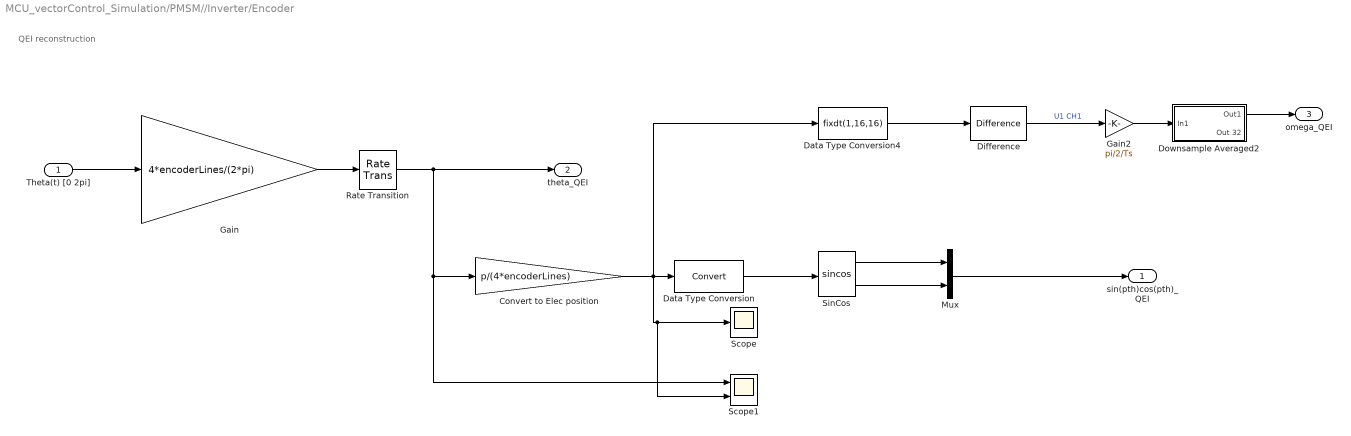
== system MCU_vectorControl_Simulation/PMSM//Inverter/Encoder ==
  note: QEI reconstruction
  Theta(t) [0 2pi] : Inport
  Convert to Elec position : Gain  Gain=p/(4*encoderLines)  ParamMax=p/(4*encoderLines)  ParamDataTypeStr=fixdt(0,16)  OutDataTypeStr=fixdt(0,16,16)
  Data Type Conversion : DataTypeConversion  SaturateOnIntegerOverflow=off  RndMeth=Floor
  Data Type Conversion4 : DataTypeConversion  OutDataTypeStr=fixdt(1,16,16)  ConvertRealWorld=Stored Integer (SI)  SaturateOnIntegerOverflow=off  RndMeth=Floor
  Difference : simulink/Discrete/Difference  ICPrevInput=0  OutMin=[]  OutMax=[]  OutDataType=fixdt(1, 16)  OutScaling=2^-10  DoSatur=off
  Downsample Averaged2 : Subsystem  mask{DownSample=10}
      mask prompts: DownSample "DownSample Factor"
  Gain : Gain  Gain=4*encoderLines/(2*pi)  OutDataTypeStr=int16
  Gain2 : Gain  Gain=pi/2/Ts  ParamMax=2*pi/4/Ts  ParamDataTypeStr=fixdt(1,16)  OutMax=pmsm.omegaMax  OutDataTypeStr=fixdt(1,16)
  Mux : Mux  Inputs=2
  Rate Transition : RateTransition  OutPortSampleTime=Ts
  Scope : Scope
  Scope1 : Scope  NumInputPorts=2
  SinCos : Trigonometry  Operator=sincos  ApproximationMethod=Lookup  AngleUnit=revolution  TableDataTypeStr=fixdt(1,16,14)
  sin(pth)cos(pth)_QEI : Outport  Unit=rad/s  VectorParamsAs1DForOutWhenUnconnected=off
  theta_QEI : Outport  Port=2
  omega_QEI : Outport  Port=3
  wires:
  Downsample Averaged2/1(Out1) -> omega_QEI/1
  Gain2/1 -> Downsample Averaged2/1(In1)
  Difference/1 -> Gain2/1  "U1 CH1"
  Data Type Conversion/1 -> SinCos/1
  Data Type Conversion4/1 -> Difference/1
  Convert to Elec position/1 -> Scope1/2, Scope/1, Data Type Conversion/1, Data Type Conversion4/1
  SinCos/1 -> Mux/1
  SinCos/2 -> Mux/2
  Mux/1 -> sin(pth)cos(pth)_QEI/1
  Rate Transition/1 -> theta_QEI/1, Scope1/1, Convert to Elec position/1
  Gain/1 -> Rate Transition/1
  Theta(t) [0 2pi]/1 -> Gain/1

== system MCU_vectorControl_Simulation/PMSM//Inverter/Inverter Average Model ==
  note: $v_{abc} = \frac{V_{dc}}{3}\underbrace{\left[\begin{array}{ccc}2&-1&-1\\-1&2&-1\\-1&-1&2 \end{array}\right]}_{M}s_{abc}$
  sabc [0 1] : Inport
  Constant : Constant  Value=Vdc
  DAC & Quantification : Subsystem
  Gain : Gain  Gain=1/3
  M : Gain  Gain=[2 -1 -1;-1 2 -1;-1 -1 2]  Multiplication=Matrix(K*u)
  Product : Product
  Saturation : Saturate  UpperLimit=1  LowerLimit=0
  "vabc (V) " : Outport  VectorParamsAs1DForOutWhenUnconnected=off
  Vdc : Outport  Port=2  VectorParamsAs1DForOutWhenUnconnected=off
  wires:
  Saturation/1 -> M/1
  Gain/1 -> "vabc (V) "/1
  Product/1 -> Gain/1
  M/1 -> Product/2
  sabc [0 1]/1 -> DAC & Quantification/1(PWM(k))
  DAC & Quantification/1(vabc(t)) -> Saturation/1
  Constant/1 -> Vdc/1, Product/1

== system MCU_vectorControl_Simulation/PMSM//Inverter/Mechanical Dynamics ==
  tau_m : Inport
  tau_l : Inport  Port=2
  Gain : Gain  Gain=1/J
  Gain1 : Gain  Gain=F
  Gain2 : Gain  Gain=C0
  Integrator : Integrator
  Integrator5 : Integrator
  Modulo by Constant2 : embmathops/Modulo by Constant  Denominator=2*pi  SimulateUsing=Code generation
  Sign : Signum
  Subtract1 : Sum  Inputs=+---
  Theta : Outport  VectorParamsAs1DForOutWhenUnconnected=off
  Omega : Outport  Port=2  VectorParamsAs1DForOutWhenUnconnected=off
  wires:
  Gain1/1 -> Subtract1/2
  Integrator/1 -> Modulo by Constant2/1
  Subtract1/1 -> Integrator5/1
  tau_l/1 -> Subtract1/4
  Integrator5/1 -> Gain/1
  Gain2/1 -> Subtract1/3
  Sign/1 -> Gain2/1
  tau_m/1 -> Subtract1/1
  Modulo by Constant2/1 -> Theta/1
  Gain/1 -> Omega/1, Gain1/1, Sign/1, Integrator/1

== system MCU_vectorControl_Simulation/Park/Clarke ==
  note: Clark transform
      | $x_{\alpha\beta} = \frac{2}{3}\underbrace{\left[\begin{array}{ccc}1&-\frac{1}{2}&-\frac{1}{2}\\0&\frac{\sqrt{3}}{2}&-\frac{\sqrt{3}}{2}\end{array}\right]}_{C_{23}}x_{abc}$
      | if only 2 currents are measured since $x_a+x_b+x_c = 0$
      | $x_{abc} = \left[\begin{array}{cc}1 & 0\\0 & 1\\-1&-1\end{array}\right]x_{ab}$
      | leading to
      | $x_{\alpha\beta} = \underbrace{\left[\begin{array}{cc}1&0\\\frac{1}{\sqrt{3}}&\frac{2}{\sqrt{3}}\end{array}\right]}_{C_{22}}x_{ab}$
  xab(c) : Inport
  C1 : Gain  Gain=[1/sqrt(3) 2/sqrt(3)]  Multiplication=Matrix(K*u)  OutDataTypeStr=Inherit: Same as input
  Mux : Mux  Inputs=2
  Selector : Selector  InputPortWidth=2  IndexOptions=Index vector (dialog)  Indices=[1]  OutputSizes=1
  xalphabeta : Outport  VectorParamsAs1DForOutWhenUnconnected=off
  wires:
  C1/1 -> Mux/2
  Selector/1 -> Mux/1
  Mux/1 -> xalphabeta/1
  xab(c)/1 -> C1/1, Selector/1

== system MCU_vectorControl_Simulation/Park/Park ==
  note: Park
      | $x_{dq} = P(\theta)^{-1}x_{\alpha\beta}\\ P(p\theta)^{-1} = \left[\begin{array}{cc}\cos(p\theta) & \sin(p\theta)\\ -\sin(p\theta) & \cos(p\theta) \end{array}\right]$
  xalphabeta : Inport  PortDimensions=2
  P(pth) : Inport  Port=2
  Data Type Duplicate2 : DataTypeDuplicate
  Park : Product  Multiplication=Matrix(*)  OutDataTypeStr=Inherit: Inherit via back propagation  RndMeth=Round
  xdq : Outport  VectorParamsAs1DForOutWhenUnconnected=off
  wires:
  P(pth)/1 -> Park/1
  xalphabeta/1 -> Park/2, Data Type Duplicate2/2
  Park/1 -> xdq/1, Data Type Duplicate2/1

== system MCU_vectorControl_Simulation/Park inverse/Clarke Inverse ==
  note: Clarke inverse
  xalphabeta : Inport
  C23' : Gain  Gain=|  Multiplication=Matrix(K*u)  OutDataTypeStr=Inherit: Inherit via back propagation  RndMeth=Round
      | [1   -1/2        -1/2;
      |         0   sqrt(3)/2   -sqrt(3)/2]'
  xabc : Outport  VectorParamsAs1DForOutWhenUnconnected=off
  wires:
  xalphabeta/1 -> C23'/1
  C23'/1 -> xabc/1

== system MCU_vectorControl_Simulation/Park inverse/Park inverse ==
  note: Inverse Park
      | $x_{\alpha\beta} = P(p\theta)x_{dq}\\ P(p\theta) = \left[\begin{array}{cc}\cos(p\theta) & -\sin(p\theta)\\ \sin(p\theta) & \cos(p\theta) \end{array}\right]$
  xdq : Inport
  P(pth) : Inport  Port=2
  Data Type Duplicate2 : DataTypeDuplicate
  Transpose : Math  Operator=transpose
  Transpose1 : Math  Operator=transpose
  xalpha sin(pth)1 : Product  Multiplication=Matrix(*)  OutDataTypeStr=Inherit: Inherit via back propagation  RndMeth=Round
  xalpahbeta : Outport  VectorParamsAs1DForOutWhenUnconnected=off
  wires:
  P(pth)/1 -> xalpha sin(pth)1/2
  Transpose1/1 -> xalpahbeta/1
  Transpose/1 -> Data Type Duplicate2/2, xalpha sin(pth)1/1
  xdq/1 -> Transpose/1
  xalpha sin(pth)1/1 -> Data Type Duplicate2/1, Transpose1/1

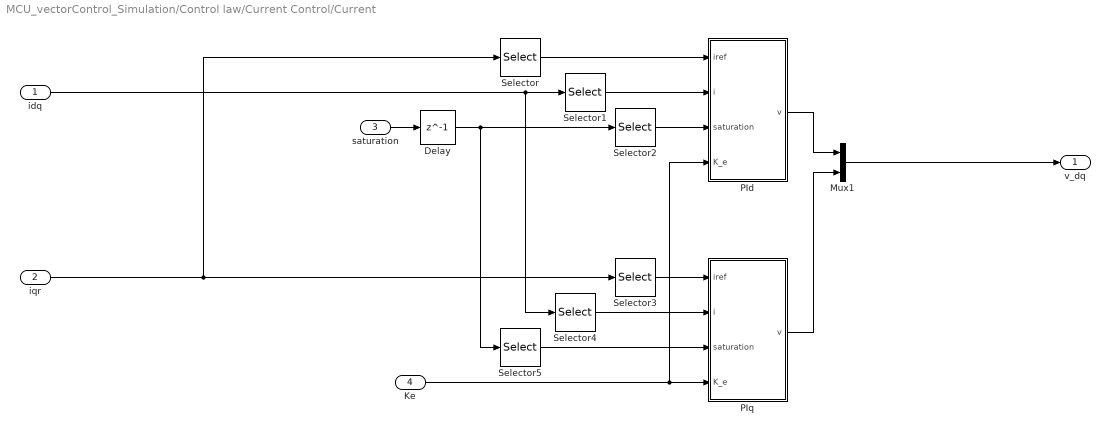
== system MCU_vectorControl_Simulation/Control law/Current Control/Current ==
  idq : Inport
  iqr : Inport  Port=2
  saturation : Inport  Port=3
  Ke : Inport  Port=4
  Delay : Delay  DelayLength=1
  Mux1 : Mux  Inputs=2
  PId : Subsystem
  PIq : Subsystem
  Selector : Selector  InputPortWidth=2  IndexOptions=Index vector (dialog)  Indices=[1]  OutputSizes=1
  Selector1 : Selector  InputPortWidth=2  IndexOptions=Index vector (dialog)  Indices=[1]  OutputSizes=1
  Selector2 : Selector  InputPortWidth=2  IndexOptions=Index vector (dialog)  Indices=[1]  OutputSizes=1
  Selector3 : Selector  InputPortWidth=2  IndexOptions=Index vector (dialog)  Indices=[2]  OutputSizes=1
  Selector4 : Selector  InputPortWidth=2  IndexOptions=Index vector (dialog)  Indices=[2]  OutputSizes=1
  Selector5 : Selector  InputPortWidth=2  IndexOptions=Index vector (dialog)  Indices=[2]  OutputSizes=1
  v_dq : Outport  VectorParamsAs1DForOutWhenUnconnected=off
  wires:
  saturation/1 -> Delay/1
  PIq/1(v) -> Mux1/2
  PId/1(v) -> Mux1/1
  idq/1 -> Selector4/1, Selector1/1
  Selector1/1 -> PId/2(i)
  Selector4/1 -> PIq/2(i)
  Mux1/1 -> v_dq/1
  Ke/1 -> PId/4(K_e), PIq/4(K_e)
  Delay/1 -> Selector5/1, Selector2/1
  Selector2/1 -> PId/3(saturation)
  Selector5/1 -> PIq/3(saturation)
  iqr/1 -> Selector3/1, Selector/1
  Selector/1 -> PId/1(iref)
  Selector3/1 -> PIq/1(iref)

== system MCU_vectorControl_Simulation/Control law/Current Control/Voltage Saturation ==
  vdq : Inport
  Divide : Product  Inputs=*/
  Gain : Gain  Gain=24/sqrt(3)
  Norm L2 : Subsystem
  Sum : Sum  Inputs=|+-
  Switch : Switch  Criteria=u2 > Threshold  Threshold=24/sqrt(3)  SaturateOnIntegerOverflow=off  InputSameDT=off
  vdqsat : Outport  VectorParamsAs1DForOutWhenUnconnected=off
  saturation : Outport  Port=2  VectorParamsAs1DForOutWhenUnconnected=off
  wires:
  Sum/1 -> saturation/1
  vdq/1 -> Switch/3, Sum/1, Divide/1, Norm L2/1(In1)
  Switch/1 -> vdqsat/1, Sum/2
  Divide/1 -> Gain/1
  Norm L2/1(y) -> Switch/2, Divide/2
  Gain/1 -> Switch/1

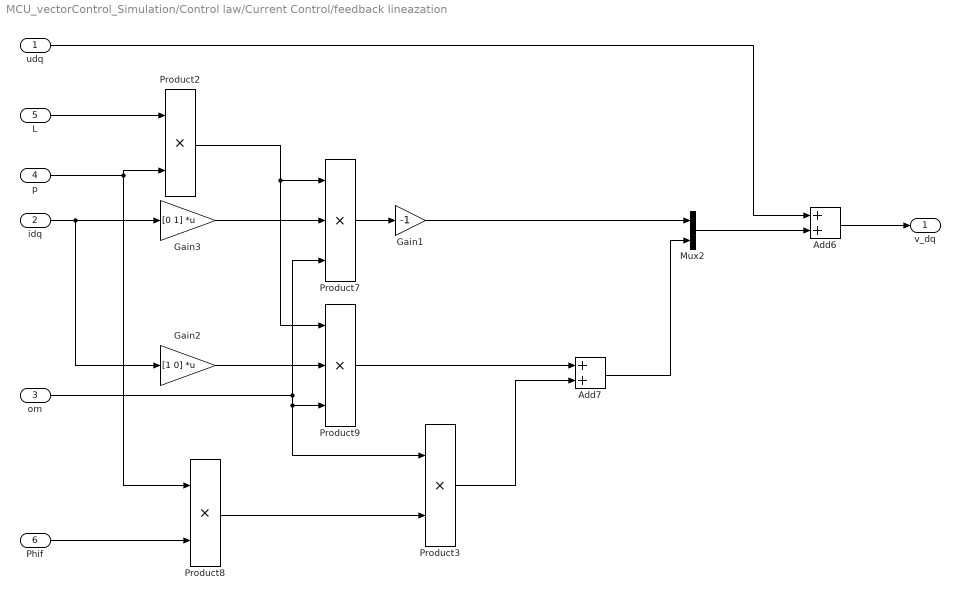
== system MCU_vectorControl_Simulation/Control law/Current Control/feedback lineazation ==
  udq : Inport
  idq : Inport  Port=2
  om : Inport  Port=3
  p : Inport  Port=4
  L : Inport  Port=5
  Phif : Inport  Port=6
  Add6 : Sum
  Add7 : Sum
  Gain1 : Gain  Gain=-1
  Gain2 : Gain  Gain=[1 0]  Multiplication=Matrix(K*u)
  Gain3 : Gain  Gain=[0 1]  Multiplication=Matrix(K*u)
  Mux2 : Mux  Inputs=2
  Product2 : Product
  Product3 : Product
  Product7 : Product  Inputs=3
  Product8 : Product
  Product9 : Product  Inputs=3
  v_dq : Outport  VectorParamsAs1DForOutWhenUnconnected=off
  wires:
  Product3/1 -> Add7/2
  Product9/1 -> Add7/1
  Gain2/1 -> Product9/2
  om/1 -> Product3/1, Product9/3, Product7/3
  Product8/1 -> Product3/2
  Phif/1 -> Product8/2
  Product7/1 -> Gain1/1
  Gain3/1 -> Product7/2
  Product2/1 -> Product7/1, Product9/1
  L/1 -> Product2/1
  p/1 -> Product2/2, Product8/1
  Gain1/1 -> Mux2/1
  idq/1 -> Gain2/1, Gain3/1
  Add6/1 -> v_dq/1
  udq/1 -> Add6/1
  Add7/1 -> Mux2/2
  Mux2/1 -> Add6/2

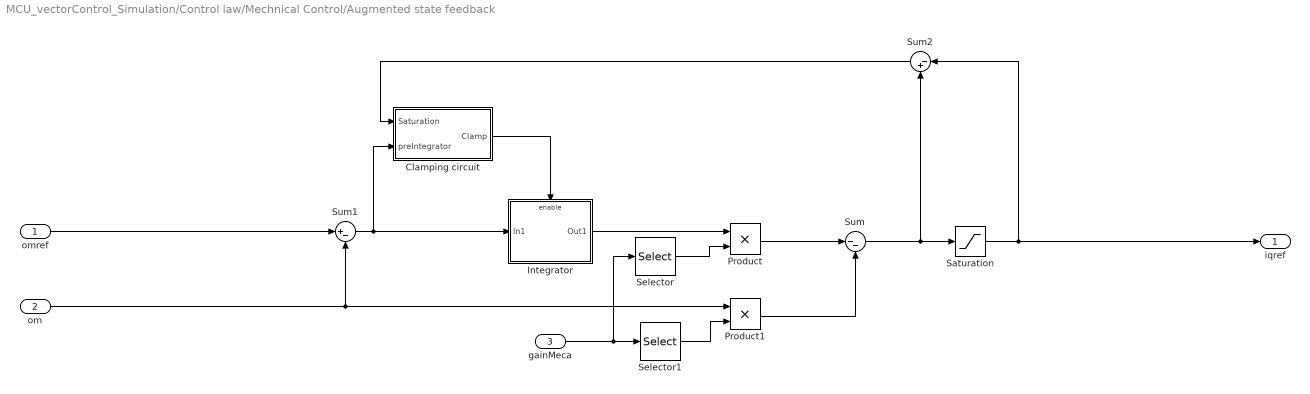
== system MCU_vectorControl_Simulation/Control law/Mechnical Control/Augmented state feedback ==
  omref : Inport
  om : Inport  Port=2
  gainMeca : Inport  Port=3
  Clamping circuit : Subsystem
  Integrator : Subsystem
  Product : Product
  Product1 : Product
  Saturation : Saturate  UpperLimit=4  LowerLimit=-4
  Selector : Selector  InputPortWidth=2  IndexOptions=Index vector (dialog)  Indices=[2]  OutputSizes=1
  Selector1 : Selector  InputPortWidth=2  IndexOptions=Index vector (dialog)  Indices=1  OutputSizes=1
  Sum : Sum  Inputs=|--  OutDataTypeStr=single  SaturateOnIntegerOverflow=on
  Sum1 : Sum  Inputs=|+-
  Sum2 : Sum  Inputs=|-+  OutDataTypeStr=Inherit: Same as accumulator  SaturateOnIntegerOverflow=on
  iqref : Outport  VectorParamsAs1DForOutWhenUnconnected=off
  wires:
  Sum/1 -> Sum2/2, Saturation/1
  Product1/1 -> Sum/2
  Product/1 -> Sum/1
  om/1 -> Sum1/2, Product1/1
  Sum1/1 -> Integrator/1(In1), Clamping circuit/2(preIntegrator)
  omref/1 -> Sum1/1
  Clamping circuit/1(Clamp) -> Integrator/Enable
  Sum2/1 -> Clamping circuit/1(Saturation)
  Integrator/1(Out1) -> Product/1
  Saturation/1 -> Sum2/1, iqref/1
  Selector1/1 -> Product1/2
  Selector/1 -> Product/2
  gainMeca/1 -> Selector1/1, Selector/1

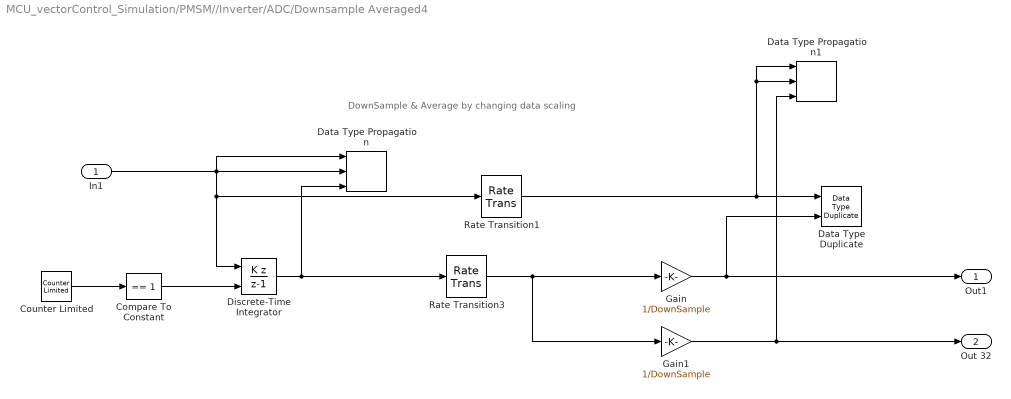
== system MCU_vectorControl_Simulation/PMSM//Inverter/ADC/Downsample Averaged4 ==
  note: DownSample & Average by changing data scaling
  In1 : Inport
  Compare To Constant : simulink/Logic and Bit Operations/Compare To Constant  relop===  const=1  OutDataTypeStr=boolean
  Counter Limited : simulink/Sources/Counter Limited  uplimit=DownSample-1  tsamp=-1
  Data Type Duplicate : DataTypeDuplicate
  Data Type Propagation : simulink/Signal Attributes/Data Type Propagation  PropDataType=fixdt(1, 16)  IfRefDouble=double  IfRefSingle=single  IsSigned=IsSigned1 or IsSigned2  NumBitsBase=NumBits1+NumBits2  NumBitsMult=1  NumBitsAdd=0  NumBitsAllowFinal=1:128  PropScaling=2^-10  ValuesUsedBestPrec=[5 -7]  SlopeBase=Slope1  SlopeMult=1  SlopeAdd=0  BiasBase=Bias1  BiasMult=1  BiasAdd=0
  Data Type Propagation1 : simulink/Signal Attributes/Data Type Propagation  PropDataType=fixdt(1, 16)  IfRefDouble=double  IfRefSingle=single  IsSigned=IsSigned1 or IsSigned2  NumBitsBase=NumBits1+NumBits2  NumBitsMult=1  NumBitsAdd=0  NumBitsAllowFinal=1:128  PropScaling=2^-10  ValuesUsedBestPrec=[5 -7]  SlopeBase=PosRange1  SlopeMult=1  SlopeAdd=0  BiasBase=Bias1  BiasMult=1  BiasAdd=0
  Discrete-Time Integrator : DiscreteIntegrator  IntegratorMethod=Accumulation: Backward Euler  gainval=1  ExternalReset=sampled level  SampleTime=-1  OutDataTypeStr=Inherit: Inherit via back propagation  ICPrevOutput=DiscIntNeverNeededParam  ICPrevScaledInput=DiscIntNeverNeededParam
  Gain : Gain  Gain=1/DownSample  OutDataTypeStr=Inherit: Inherit via back propagation  RndMeth=Round
  Gain1 : Gain  Gain=1/DownSample  OutDataTypeStr=Inherit: Inherit via back propagation
  Rate Transition1 : RateTransition  OutPortSampleTimeOpt=Multiple of input port sample time  OutPortSampleTimeMultiple=DownSample  OutPortSampleTime=DownSample
  Rate Transition3 : RateTransition  OutPortSampleTimeOpt=Multiple of input port sample time  OutPortSampleTimeMultiple=DownSample  OutPortSampleTime=DownSample
  Out1 : Outport  VectorParamsAs1DForOutWhenUnconnected=off
  Out 32 : Outport  Port=2  VectorParamsAs1DForOutWhenUnconnected=off
  wires:
  Gain1/1 -> Data Type Propagation1/3, Out 32/1
  Rate Transition1/1 -> Data Type Duplicate/1, Data Type Propagation1/1, Data Type Propagation1/2
  Gain/1 -> Out1/1, Data Type Duplicate/2
  Counter Limited/1 -> Compare To Constant/1
  Discrete-Time Integrator/1 -> Rate Transition3/1, Data Type Propagation/3
  Compare To Constant/1 -> Discrete-Time Integrator/2
  In1/1 -> Data Type Propagation/1, Data Type Propagation/2, Discrete-Time Integrator/1, Rate Transition1/1
  Rate Transition3/1 -> Gain/1, Gain1/1

== system MCU_vectorControl_Simulation/PMSM//Inverter/Dead Time Modeling/DeadTime Compensation ==
  note: Deat Time Compensation
  iabc : Inport
  Enable : EnablePort  StatesWhenEnabling=reset
  Gain1 : Gain  Gain=dT*1e-6*FPWM
  Gain2 : Gain  Gain=Vdc
  Sign : Signum
  Delta vabc : Outport
  wires:
  Sign/1 -> Gain1/1
  Gain1/1 -> Gain2/1
  Gain2/1 -> Delta vabc/1
  iabc/1 -> Sign/1
